simulink model "ESPSIM_Reception_Multiplex"  (R2025a)
settings: Solver=ode3  StartTime=0.0  StopTime=inf  RelTol=1e-3  EnableMultiTasking=on
libraries: simulink x6, arduinolib x3
settings Model: FPTRunName=Active  SimulationMode=external  SILPILModeSetting=veronly  ExtModeTrigDuration=2  Creator=antho  LastModifiedBy=antho
settings SolverCC: AlgebraicLoopSolver=TrustRegion  AutoInsertRateTranBlk=on
settings DataIOCC: LimitDataPoints=on  SaveFormat=Array
settings OptimizationCC: ReuseModelBlockBuffer=off  ExpressionDepthLimit=2147483647.0  LifeSpan=Inf  MaxStackSize=64
settings DebuggingCC: UnderspecifiedInitializationDetection=Classic  MergeDetectMultiDrivingBlocksExec=none  FcnCallInpInsideContextMsg=warning  UnconnectedInputMsg=warning  UnconnectedOutputMsg=warning  UnconnectedLineMsg=warning  AllowSymbolicDim=off  StateNameClashWarn=warning  SFUnexpectedBacktrackingDiag=warning  SFNoUnconditionalDefaultTransitionDiag=warning  SFExecutionAtInitializationDiag=none  ArithmeticOperatorsInVariantConditions=warning
settings HardwareCC: ProdBitPerPointer=32.0  ProdBitPerSizeT=32.0  ProdBitPerPtrDiffT=32.0  ProdLargestAtomicInteger=Long  ProdLargestAtomicFloat=Double  ProdWordSize=32.0  ProdHWDeviceType=ARM Compatible->ARM Cortex
settings ModelReferenceCC: EnableRefExpFcnMdlSchedulingChecks=on  PropagateSignalLabelsOutOfModel=off
settings SFSimCC: SimUseLocalCustomCode=off  CustomCodeUndefinedFunction=UseInterfaceOnly
settings RTWCC: SystemTargetFile=ert.tlc  HardwareBoard=ESP32-WROOM (Arduino Compatible)  TemplateMakefile=ert_default_tmf  GenerateReport=on  RTWVerbose=off  RTWUseLocalCustomCode=off  Toolchain=ESP32  BuildConfiguration=Faster Runs  LaunchReport=on  GPUComputeCapability=3.5  Description=Embedded Coder
settings CodeAppCC: ForceParamTrailComments=on  OperatorAnnotations=on  StateflowObjectComments=on  MATLABSourceComments=on
settings ERTTargetCC: ExtModeTransport=3.0  ExtModeAutomaticAllocSize=off  ExtModeStaticAllocSize=65536.0  InlinedParameterPlacement=Hierarchical  DynamicArrayContainerType=coder::array  MultiwordLength=2048.0  ERTCustomFileBanners=off  SupportContinuousTime=on  SupportNonInlinedSFcns=on  RemoveResetFunc=off  SupportVariableSizeSignals=on  ModelStepFunctionPrototypeControlCompliant=off
settings ConfigComp: CovMetricSettings=dw  CovSaveCumulativeToWorkspaceVar=on  CovSaveSingleToWorkspaceVar=on  CovExternalEMLEnable=off  CovSFcnEnable=off

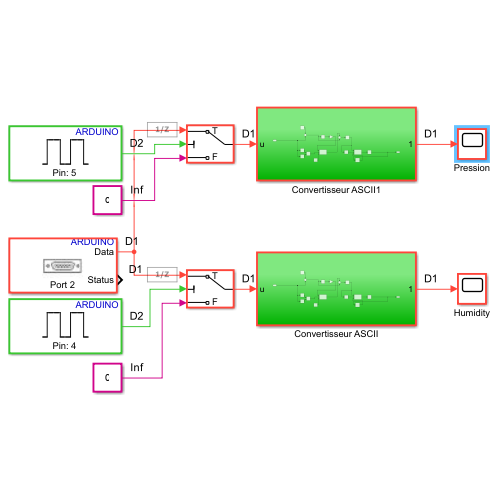
[thumbnail: Simulink's stored preview of the top-level diagram]
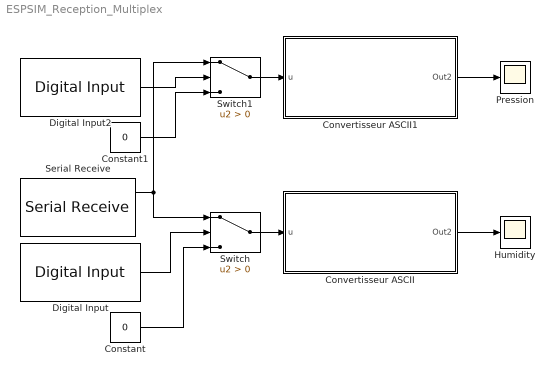
== system ESPSIM_Reception_Multiplex ==
  Constant : Constant  Value=0
  Constant1 : Constant  Value=0
  Convertisseur ASCII : Subsystem
  Convertisseur ASCII1 : Subsystem
  Digital Input : arduinolib/Digital Input  pinNumber=4  mode=Default  Direction=input  SampleTime=0.1  blockPlatform=arduino
  Digital Input2 : arduinolib/Digital Input  pinNumber=5  mode=Default  Direction=input  SampleTime=0.1  blockPlatform=arduino
  Humidity : Scope
      settings: ActiveDisplayYMinimum=-12.374999999999996  ActiveDisplayYMaximum=111.375  DataLoggingVariableName=ScopeData4
  Pression : Scope
      settings: ActiveDisplayYMinimum=-12.374999999999996  ActiveDisplayYMaximum=111.375
  Serial Receive : arduinolib/Serial Receive  portNumber=2  DataType=uint8  blockPlatform=ARDUINO  TimeOut=0  MaxDataLength=10  isARMArch=off  DataLengthOption=Length via dialog  Datalength=1  Header=[]  Terminator=[]  SampleTime=0.01  ShowOutStatus=on
  Switch : Switch  Criteria=u2 > Threshold  SaturateOnIntegerOverflow=off  InputSameDT=off
  Switch1 : Switch  Criteria=u2 > Threshold  SaturateOnIntegerOverflow=off  InputSameDT=off
  wires:
  Convertisseur ASCII/1(Out2) -> Humidity/1
  Constant/1 -> Switch/3
  Digital Input/1 -> Switch/2
  Switch/1 -> Convertisseur ASCII/1(u)
  Serial Receive/1 -> Switch/1, Switch1/1
  Switch1/1 -> Convertisseur ASCII1/1(u)
  Digital Input2/1 -> Switch1/2
  Constant1/1 -> Switch1/3
  Convertisseur ASCII1/1(Out2) -> Pression/1

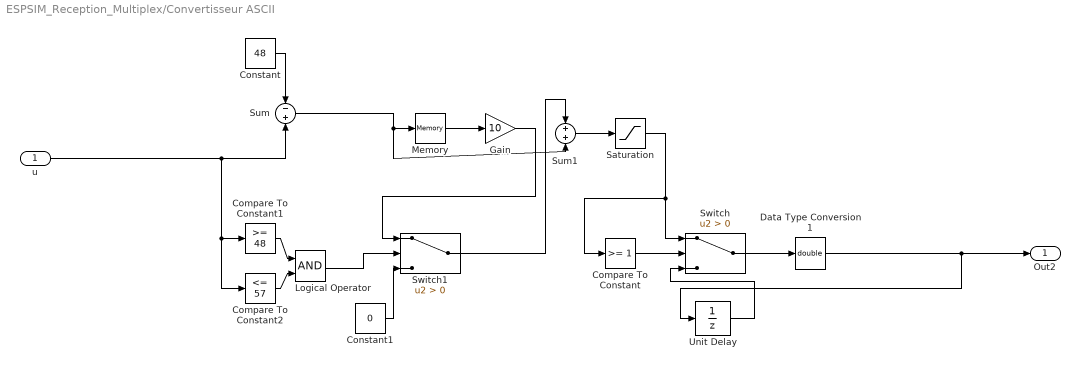
== system ESPSIM_Reception_Multiplex/Convertisseur ASCII ==
  u : Inport
  Compare To Constant : simulink/Logic and Bit Operations/Compare To Constant  relop=>=  const=1  OutDataTypeStr=boolean
  Compare To Constant1 : simulink/Logic and Bit Operations/Compare To Constant  relop=>=  const=48  OutDataTypeStr=boolean
  Compare To Constant2 : simulink/Logic and Bit Operations/Compare To Constant  relop=<=  const=57  OutDataTypeStr=boolean
  Constant : Constant  Value=48
  Constant1 : Constant  Value=0
  Data Type Conversion1 : DataTypeConversion  OutDataTypeStr=double  SaturateOnIntegerOverflow=off  RndMeth=Floor
  Gain : Gain  Gain=10
  Logical Operator : Logic  AllPortsSameDT=off  OutDataTypeStr=boolean
  Memory : Memory  InheritSampleTime=on  LinearizeAsDelay=on
  Saturation : Saturate  UpperLimit=100  LowerLimit=0  OutDataTypeStr=double
  Sum : Sum  Inputs=-+
  Sum1 : Sum
  Switch : Switch  Criteria=u2 > Threshold  SaturateOnIntegerOverflow=off  InputSameDT=off
  Switch1 : Switch  Criteria=u2 > Threshold  SaturateOnIntegerOverflow=off  InputSameDT=off
  Unit Delay : UnitDelay  SampleTime=-1  HasFrameUpgradeWarning=on
  Out2 : Outport
  wires:
  u/1 -> Sum/2, Compare To Constant1/1, Compare To Constant2/1
  Switch1/1 -> Sum1/1
  Sum/1 -> Sum1/2, Memory/1
  Constant/1 -> Sum/1
  Unit Delay/1 -> Switch/3
  Memory/1 -> Gain/1
  Compare To Constant/1 -> Switch/2
  Sum1/1 -> Saturation/1
  Saturation/1 -> Switch/1, Compare To Constant/1
  Compare To Constant1/1 -> Logical Operator/1
  Data Type Conversion1/1 -> Out2/1, Unit Delay/1
  Switch/1 -> Data Type Conversion1/1
  Constant1/1 -> Switch1/3
  Logical Operator/1 -> Switch1/2
  Compare To Constant2/1 -> Logical Operator/2
  Gain/1 -> Switch1/1

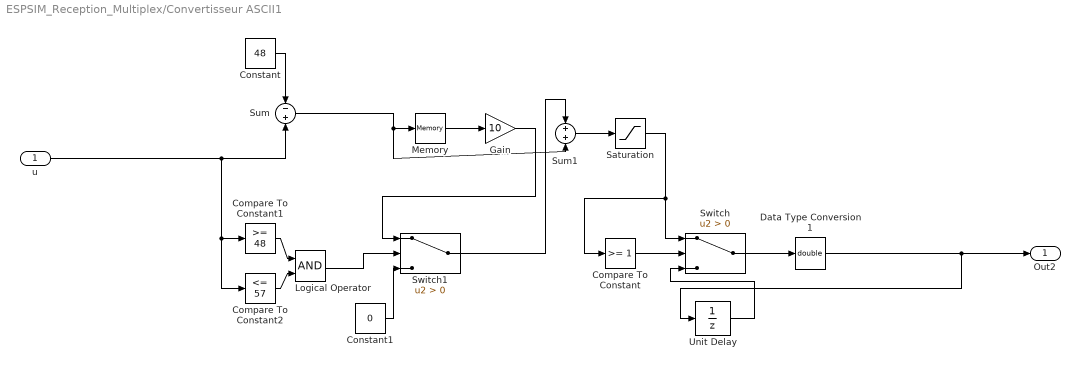
== system ESPSIM_Reception_Multiplex/Convertisseur ASCII1 ==
  u : Inport
  Compare To Constant : simulink/Logic and Bit Operations/Compare To Constant  relop=>=  const=1  OutDataTypeStr=boolean
  Compare To Constant1 : simulink/Logic and Bit Operations/Compare To Constant  relop=>=  const=48  OutDataTypeStr=boolean
  Compare To Constant2 : simulink/Logic and Bit Operations/Compare To Constant  relop=<=  const=57  OutDataTypeStr=boolean
  Constant : Constant  Value=48
  Constant1 : Constant  Value=0
  Data Type Conversion1 : DataTypeConversion  OutDataTypeStr=double  SaturateOnIntegerOverflow=off  RndMeth=Floor
  Gain : Gain  Gain=10
  Logical Operator : Logic  AllPortsSameDT=off  OutDataTypeStr=boolean
  Memory : Memory  InheritSampleTime=on  LinearizeAsDelay=on
  Saturation : Saturate  UpperLimit=100  LowerLimit=0  OutDataTypeStr=double
  Sum : Sum  Inputs=-+
  Sum1 : Sum
  Switch : Switch  Criteria=u2 > Threshold  SaturateOnIntegerOverflow=off  InputSameDT=off
  Switch1 : Switch  Criteria=u2 > Threshold  SaturateOnIntegerOverflow=off  InputSameDT=off
  Unit Delay : UnitDelay  SampleTime=-1  HasFrameUpgradeWarning=on
  Out2 : Outport
  wires:
  u/1 -> Sum/2, Compare To Constant1/1, Compare To Constant2/1
  Switch1/1 -> Sum1/1
  Sum/1 -> Sum1/2, Memory/1
  Constant/1 -> Sum/1
  Unit Delay/1 -> Switch/3
  Memory/1 -> Gain/1
  Compare To Constant/1 -> Switch/2
  Sum1/1 -> Saturation/1
  Saturation/1 -> Switch/1, Compare To Constant/1
  Compare To Constant1/1 -> Logical Operator/1
  Data Type Conversion1/1 -> Out2/1, Unit Delay/1
  Switch/1 -> Data Type Conversion1/1
  Constant1/1 -> Switch1/3
  Logical Operator/1 -> Switch1/2
  Compare To Constant2/1 -> Logical Operator/2
  Gain/1 -> Switch1/1
